simulink model "qu_sim"  (R2020b)
settings: Solver=FixedStepAuto  StartTime=0.0  StopTime=100  FixedStep=0.0001  RelTol=1e-3
undefined symbols (not defined in the file or in its folder): m, n
settings Model: Creator=Bennu  LastModifiedBy=Bennu
settings DataIOCC: SaveOutput=off  SaveTime=off  ReturnWorkspaceOutputs=off
settings DebuggingCC: ArithmeticOperatorsInVariantConditions=warning
settings SFSimCC: SimUseLocalCustomCode=off  CustomCodeUndefinedFunction=UseInterfaceOnly
settings RTWCC: RTWUseLocalCustomCode=off
settings CodeAppCC: StateflowObjectComments=on

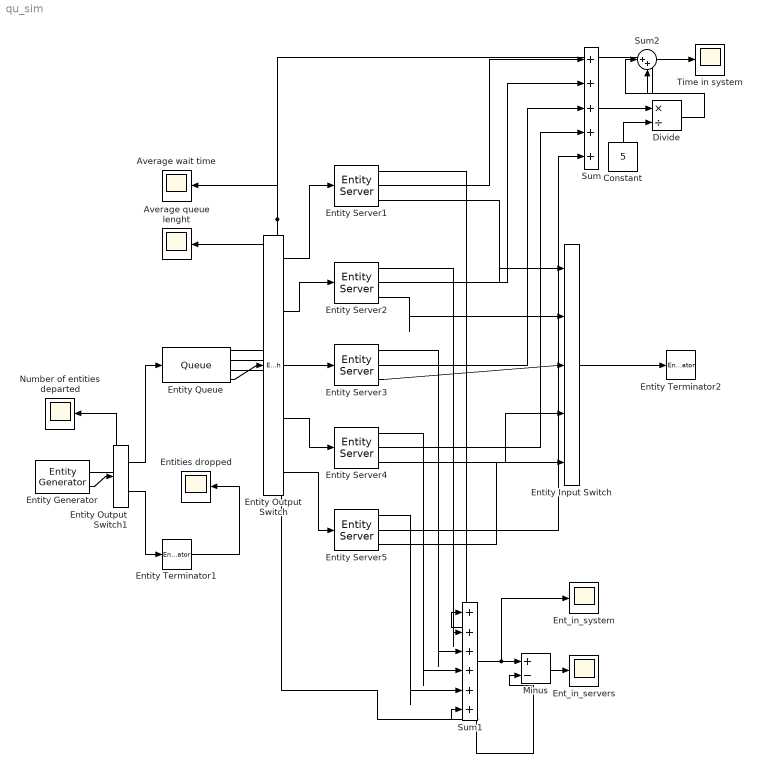
== system qu_sim ==
  Average queue lenght : Scope
  Average wait time : Scope
  Constant : Constant  Value=5
  Divide : Product  Inputs=*/
  Ent_in_servers : Scope
  Ent_in_system : Scope
  Entities dropped : Scope
  Entity Input Switch : EntityInputSwitch  InputPortMessageModes=m,m,m,m,m  OutputPortMessageModes=m  NumberInputPorts=5
      settings: InputPortMap=u1,u2,u3,u4,u5
  Entity Output Switch : EntityOutputSwitch  InputPortMessageModes=m  OutputPortMessageModes=m,m,m,m,m  NumberOutputPorts=5  SwitchAttributeName=Attribute1
      settings: OutputPortMap=o0,o1,o2,o3,o4
  Entity Output Switch1 : EntityOutputSwitch  InputPortMessageModes=m  OutputPortMessageModes=m,m  SwitchAttributeName=Attribute1
  Entity Generator : EntityGenerator  OutputPortMessageModes=n,m  TimeSource=MATLAB action  IntergenerationTimeAction=|  GenerateEntityAtSimulationStart=off  GenerateAction=|  AttributeName=Number  AttributeInitialValue=0  NumberEntitiesDeparted=on  EntityType=Structured  EntityTypeName=Entity
      IntergenerationTimeAction=|
      | persistent rngInit;
      | 
      | if isempty(rngInit)
      |     seed = 123;
      |     rng(seed);
      |     rngInit = true;
      | end
      | 
      | % Pattern: Exponential distribution
      | lambda = 460;
      | dt = -(1/lambda)*log(1-rand());
      GenerateAction=|
      | % Pattern: Repeating Sequence
      | 
      | persistent idx;
      | idx = 1;
      | entity.Number = idx;
      | 
      | coder.extrinsic('assignin');
      | idx = idx + 1;
      settings: OutputPortMap=o0,o3
  Entity Queue : Queue  InputPortMessageModes=m  OutputPortMessageModes=n,n,n,m  Capacity=4  NumberEntitiesInBlock=on  AverageWait=on  AverageQueueLength=on
      settings: OutputPortMap=o1,o2,o3,o5
  Entity Server1 : EntityServer  InputPortMessageModes=m  OutputPortMessageModes=n,n,m  Capacity=1  ServiceTimeSource=MATLAB action  ServiceTimeAction=|  NumberEntitiesInBlock=on  AverageWait=on
      | persistent rngInit;
      | 
      | if isempty(rngInit)
      |     seed = 213123;
      |     rng(seed);
      |     rngInit = true;
      | end
      | 
      | mu = 100;
      | dt = -(1/mu)*log(1-rand());
      settings: OutputPortMap=o1,o4,o9
  Entity Server2 : EntityServer  InputPortMessageModes=m  OutputPortMessageModes=n,n,m  Capacity=1  ServiceTimeSource=MATLAB action  ServiceTimeAction=|  NumberEntitiesInBlock=on  AverageWait=on
      | persistent rngInit;
      | 
      | if isempty(rngInit)
      |     seed = 21323;
      |     rng(seed);
      |     rngInit = true;
      | end
      | 
      | mu = 100;
      | dt = -(1/mu)*log(1-rand());
      settings: OutputPortMap=o1,o4,o9
  Entity Server3 : EntityServer  InputPortMessageModes=m  OutputPortMessageModes=n,n,m  Capacity=1  ServiceTimeSource=MATLAB action  ServiceTimeAction=|  NumberEntitiesInBlock=on  AverageWait=on
      | persistent rngInit;
      | 
      | if isempty(rngInit)
      |     seed = 3421412;
      |     rng(seed);
      |     rngInit = true;
      | end
      | 
      | mu = 100;
      | dt = -(1/mu)*log(1-rand());
      settings: OutputPortMap=o1,o4,o9
  Entity Server4 : EntityServer  InputPortMessageModes=m  OutputPortMessageModes=n,n,m  Capacity=1  ServiceTimeSource=MATLAB action  ServiceTimeAction=|  NumberEntitiesInBlock=on  AverageWait=on
      | persistent rngInit;
      | 
      | if isempty(rngInit)
      |     seed = 3532;
      |     rng(seed);
      |     rngInit = true;
      | end
      | 
      | mu = 80;
      | dt = -(1/mu)*log(1-rand());
      settings: OutputPortMap=o1,o4,o9
  Entity Server5 : EntityServer  InputPortMessageModes=m  OutputPortMessageModes=n,n,m  Capacity=1  ServiceTimeSource=MATLAB action  ServiceTimeAction=|  NumberEntitiesInBlock=on  AverageWait=on
      | persistent rngInit;
      | 
      | if isempty(rngInit)
      |     seed = 3123;
      |     rng(seed);
      |     rngInit = true;
      | end
      | 
      | mu = 80;
      | dt = -(1/mu)*log(1-rand());
      settings: OutputPortMap=o1,o4,o9
  Entity Terminator1 : EntityTerminator  InputPortMessageModes=m  NumberEntitiesArrived=on
      settings: OutputPortMap=o0
  Entity Terminator2 : EntityTerminator  InputPortMessageModes=m  NumberEntitiesArrived=on
      settings: OutputPortMap=o0
  Minus : Sum  Inputs=+-
  Number of entities departed : Scope
  Sum : Sum  Inputs=+++++
  Sum1 : Sum  Inputs=++++++
  Sum2 : Sum  Inputs=|++
  Time in system : Scope
  wires:
  Entity Generator/2 -> Entity Output Switch1/1
  Entity Generator/1 -> Number of entities departed/1
  Entity Queue/4 -> Entity Output Switch/1
  Entity Server2/3 -> Entity Input Switch/2
  Entity Output Switch/1 -> Entity Server1/1
  Entity Output Switch/2 -> Entity Server2/1
  Entity Output Switch/3 -> Entity Server3/1
  Entity Output Switch/4 -> Entity Server4/1
  Entity Server1/3 -> Entity Input Switch/1
  Entity Server3/3 -> Entity Input Switch/3
  Entity Server4/3 -> Entity Input Switch/4
  Entity Server5/3 -> Entity Input Switch/5
  Entity Output Switch/5 -> Entity Server5/1
  Entity Input Switch/1 -> Entity Terminator2/1
  Entity Server1/1 -> Sum1/1
  Entity Server2/1 -> Sum1/2
  Entity Server3/1 -> Sum1/3
  Entity Server4/1 -> Sum1/4
  Entity Server5/1 -> Sum1/5
  Entity Queue/1 -> Minus/2, Sum1/6
  Entity Output Switch1/2 -> Entity Terminator1/1
  Entity Output Switch1/1 -> Entity Queue/1
  Entity Queue/3 -> Average queue lenght/1
  Entity Terminator1/1 -> Entities dropped/1
  Entity Queue/2 -> Average wait time/1, Sum2/1
  Sum1/1 -> Minus/1, Ent_in_system/1
  Minus/1 -> Ent_in_servers/1
  Entity Server5/2 -> Sum/5
  Entity Server4/2 -> Sum/4
  Entity Server3/2 -> Sum/3
  Entity Server2/2 -> Sum/2
  Entity Server1/2 -> Sum/1
  Sum/1 -> Divide/1
  Sum2/1 -> Time in system/1
  Constant/1 -> Divide/2
  Divide/1 -> Sum2/2
